simulink model "P6s"  (R2015b)
settings: Solver=VariableStepAuto  StartTime=0.0  StopTime=10.0  RelTol=1e-3
libraries: fl_lib x26, nesl_utility x9
settings Model: Creator=xmax1946  LastModifiedBy=xmax1946

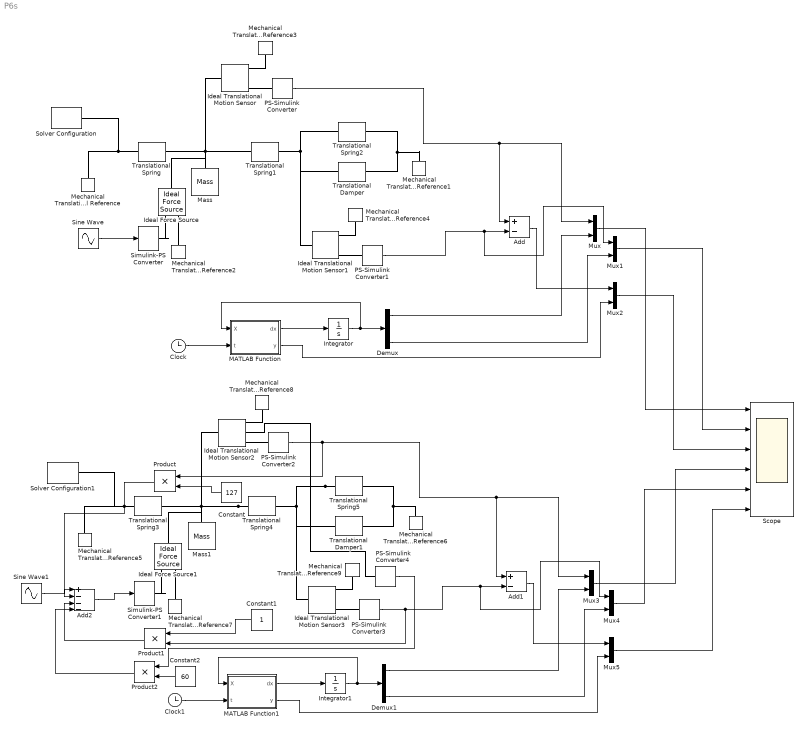
== system P6s ==
  Add : Sum  Inputs=+-
  Add1 : Sum  Inputs=+-
  Add2 : Sum  Inputs=+---
  Clock : Clock
  Clock1 : Clock
  Constant : Constant  Value=127
  Constant1 : Constant
  Constant2 : Constant  Value=60
  Demux : Demux  Outputs=3
  Demux1 : Demux  Outputs=3
  Ideal Force Source : fl_lib/Mechanical/Mechanical Sources/Ideal Force Source
  Ideal Force Source1 : fl_lib/Mechanical/Mechanical Sources/Ideal Force Source
  Ideal Translational Motion Sensor{,1..3} (4 alike) : fl_lib/Mechanical/Mechanical Sensors/Ideal Translational Motion Sensor  offset=0 m
  Integrator : Integrator  InitialCondition=[0;0;0]
  Integrator1 : Integrator  InitialCondition=[0;0;0]
  MATLAB Function : MATLAB Function  TreatAsAtomicUnit=on
  MATLAB Function1 : MATLAB Function  TreatAsAtomicUnit=on
  Mass : fl_lib/Mechanical/Translational Elements/Mass  mass=10 kg  v_specify=off  v_priority=None  v=0 m/s  f_specify=off  f_priority=None  f=0 N
  Mass1 : fl_lib/Mechanical/Translational Elements/Mass  mass=10 kg  v_specify=off  v_priority=None  v=0 m/s  f_specify=off  f_priority=None  f=0 N
  Mechanical Translational Reference{,1..9} (10 alike) : fl_lib/Mechanical/Translational Elements/Mechanical Translational Reference
  Mux{,1..5} (6 alike) : Mux  Inputs=2
  PS-Simulink Converter{,1..4} (5 alike) : nesl_utility/PS-Simulink Converter  PhysicalDomain=network_engine_domain  SubClassName=ps_output  LeftPortType=input  RightPortType=output  PseudoPeriodic=off  Frequencies=[]  Unit=1  AffineConversion=off
  Product : Product
  Product1 : Product
  Product2 : Product
  Scope : Scope  NumInputPorts=6
  Simulink-PS Converter : nesl_utility/Simulink-PS Converter  PhysicalDomain=network_engine_domain  SubClassName=ps_input  LeftPortType=input  RightPortType=output  PseudoPeriodic=off  Frequencies=[]  NoiseDistribution=none  NoiseParameters=[]  Unit=1  AffineConversion=off  InputFiltering=off  SimscapeFilterOrder=1  InputFilterTimeConstant=0.001  UdotUserProvided=1
  Simulink-PS Converter1 : nesl_utility/Simulink-PS Converter  PhysicalDomain=network_engine_domain  SubClassName=ps_input  LeftPortType=input  RightPortType=output  PseudoPeriodic=off  Frequencies=[]  NoiseDistribution=none  NoiseParameters=[]  Unit=1  AffineConversion=off  InputFiltering=off  SimscapeFilterOrder=1  InputFilterTimeConstant=0.001  UdotUserProvided=1
  Sine Wave : Sin  SampleTime=0
  Sine Wave1 : Sin  SampleTime=0
  Solver Configuration : nesl_utility/Solver Configuration  PhysicalDomain=network_engine_domain  SubClassName=solver  LeftPortType=input  RightPortType=generic  Accelerate=off  Tones=[]  Harmonics=[]  SimulateNoise=off  Profile=off  UseLocalSampling=off  EnableSwitchedLinearOptims=on  FrequencyDomain=off  UseCCode=off  RelTol=0.001  AbsTol=1e-06  MinStep=1e-09  ToWorkspace=off  RevertToSquareIcSolve=off  NumHomotopyIterations=100  PhasorMode=off  PhasorModeNumHarmonics=1  DoDC=off  ResidualTolerance=1e-09  UseLocalSolver=off  LocalSolverChoice=NE_BACKWARD_EULER_ADVANCER  LocalSolverSampleTime=0.001  DoFixedCost=off  MaxNonlinIter=3  MaxModeIter=2  LinearAlgebra=Sparse  DelaysMemoryBudget=1024  AutomaticFiltering=on  FilteringTimeConstant=0.001
  Solver Configuration1 : nesl_utility/Solver Configuration  PhysicalDomain=network_engine_domain  SubClassName=solver  LeftPortType=input  RightPortType=generic  Accelerate=off  Tones=[]  Harmonics=[]  SimulateNoise=off  Profile=off  UseLocalSampling=off  EnableSwitchedLinearOptims=on  FrequencyDomain=off  UseCCode=off  RelTol=0.001  AbsTol=1e-06  MinStep=1e-09  ToWorkspace=off  RevertToSquareIcSolve=off  NumHomotopyIterations=100  PhasorMode=off  PhasorModeNumHarmonics=1  DoDC=off  ResidualTolerance=1e-09  UseLocalSolver=off  LocalSolverChoice=NE_BACKWARD_EULER_ADVANCER  LocalSolverSampleTime=0.001  DoFixedCost=off  MaxNonlinIter=3  MaxModeIter=2  LinearAlgebra=Sparse  DelaysMemoryBudget=1024  AutomaticFiltering=on  FilteringTimeConstant=0.001
  Translational Damper : fl_lib/Mechanical/Translational Elements/Translational Damper  D=.5 N/(m/s)  v_specify=off  v_priority=None  v=0 m/s  f_specify=off  f_priority=None  f=0 N
  Translational Damper1 : fl_lib/Mechanical/Translational Elements/Translational Damper  D=.5 N/(m/s)  v_specify=off  v_priority=None  v=0 m/s  f_specify=off  f_priority=None  f=0 N
  Translational Spring : fl_lib/Mechanical/Translational Elements/Translational Spring  spr_rate=2 N/m  v_specify=off  v_priority=None  v=0 m/s  f_specify=off  f_priority=None  f=0 N  x_specify=off  x_priority=None  x=0 m
  Translational Spring1 : fl_lib/Mechanical/Translational Elements/Translational Spring  spr_rate=1 N/m  v_specify=off  v_priority=None  v=0 m/s  f_specify=off  f_priority=None  f=0 N  x_specify=off  x_priority=None  x=0 m
  Translational Spring2 : fl_lib/Mechanical/Translational Elements/Translational Spring  spr_rate=.5 N/m  v_specify=off  v_priority=None  v=0 m/s  f_specify=off  f_priority=None  f=0 N  x_specify=off  x_priority=None  x=0 m
  Translational Spring3 : fl_lib/Mechanical/Translational Elements/Translational Spring  spr_rate=2 N/m  v_specify=off  v_priority=None  v=0 m/s  f_specify=off  f_priority=None  f=0 N  x_specify=off  x_priority=None  x=0 m
  Translational Spring4 : fl_lib/Mechanical/Translational Elements/Translational Spring  spr_rate=1 N/m  v_specify=off  v_priority=None  v=0 m/s  f_specify=off  f_priority=None  f=0 N  x_specify=off  x_priority=None  x=0 m
  Translational Spring5 : fl_lib/Mechanical/Translational Elements/Translational Spring  spr_rate=.5 N/m  v_specify=off  v_priority=None  v=0 m/s  f_specify=off  f_priority=None  f=0 N  x_specify=off  x_priority=None  x=0 m
  wires:
  Sine Wave/1 -> Simulink-PS Converter/1
  PS-Simulink Converter/1 -> Mux/1, Add/1
  PS-Simulink Converter1/1 -> Mux1/1, Add/2
  MATLAB Function/1(dx) -> Integrator/1
  Integrator/1 -> MATLAB Function/1(X), Demux/1
  Clock/1 -> MATLAB Function/2(t)
  Mux/1 -> Scope/1
  Demux/1 -> Mux/2
  Mux1/1 -> Scope/2
  Demux/3 -> Mux1/2
  Mux2/1 -> Scope/3
  Add/1 -> Mux2/1
  MATLAB Function/2(y) -> Mux2/2
  PS-Simulink Converter3/1 -> Product1/2, Mux4/1, Add1/2
  MATLAB Function1/1(dx) -> Integrator1/1
  Integrator1/1 -> MATLAB Function1/1(X), Demux1/1
  Clock1/1 -> MATLAB Function1/2(t)
  Mux3/1 -> Scope/4
  Demux1/1 -> Mux3/2
  Mux4/1 -> Scope/5
  Demux1/3 -> Mux4/2
  Mux5/1 -> Scope/6
  Add1/1 -> Mux5/1
  MATLAB Function1/2(y) -> Mux5/2
  PS-Simulink Converter2/1 -> Product/1, Mux3/1, Add1/1
  Constant/1 -> Product/2
  Constant1/1 -> Product1/1
  Sine Wave1/1 -> Add2/1
  Product/1 -> Add2/2
  Product1/1 -> Add2/3
  Add2/1 -> Simulink-PS Converter1/1
  Constant2/1 -> Product2/2
  PS-Simulink Converter4/1 -> Product2/1
  Product2/1 -> Add2/4
  connections:
  Translational Spring/RConn1 -- Ideal Translational Motion Sensor/LConn1 -- Ideal Force Source/LConn1 -- Mass/LConn1 -- Translational Spring1/LConn1
  Translational Spring1/RConn1 -- Ideal Translational Motion Sensor1/LConn1 -- Translational Damper/LConn1 -- Translational Spring2/LConn1
  Mechanical Translational Reference/LConn1 -- Solver Configuration/RConn1 -- Translational Spring/LConn1
  Mechanical Translational Reference1/LConn1 -- Translational Spring2/RConn1 -- Translational Damper/RConn1
  Simulink-PS Converter/RConn1 -- Ideal Force Source/RConn1
  Mechanical Translational Reference2/LConn1 -- Ideal Force Source/RConn2
  Mechanical Translational Reference3/LConn1 -- Ideal Translational Motion Sensor/RConn1
  PS-Simulink Converter/LConn1 -- Ideal Translational Motion Sensor/RConn3
  PS-Simulink Converter1/LConn1 -- Ideal Translational Motion Sensor1/RConn3
  Mechanical Translational Reference4/LConn1 -- Ideal Translational Motion Sensor1/RConn1
  Translational Spring4/LConn1 -- Translational Spring3/RConn1 -- Ideal Translational Motion Sensor2/LConn1 -- Ideal Force Source1/LConn1 -- Mass1/LConn1
  Translational Spring5/LConn1 -- Translational Spring4/RConn1 -- Ideal Translational Motion Sensor3/LConn1 -- Translational Damper1/LConn1
  Translational Spring3/LConn1 -- Mechanical Translational Reference5/LConn1 -- Solver Configuration1/RConn1
  Translational Damper1/RConn1 -- Mechanical Translational Reference6/LConn1 -- Translational Spring5/RConn1
  Simulink-PS Converter1/RConn1 -- Ideal Force Source1/RConn1
  Mechanical Translational Reference7/LConn1 -- Ideal Force Source1/RConn2
  Mechanical Translational Reference8/LConn1 -- Ideal Translational Motion Sensor2/RConn1
  PS-Simulink Converter2/LConn1 -- Ideal Translational Motion Sensor2/RConn3
  PS-Simulink Converter3/LConn1 -- Ideal Translational Motion Sensor3/RConn3
  Mechanical Translational Reference9/LConn1 -- Ideal Translational Motion Sensor3/RConn1
  PS-Simulink Converter4/LConn1 -- Ideal Translational Motion Sensor2/RConn2

== matlab function P6s/MATLAB Function1 ==
  data: dx output; X input; y output; t input
function [dx,y] = fcn(X,t)

m1=10;
k1=2;
k2=1;
k3=.5;
b1=.5;
K=[127,60,1];
A=[0,1,0;-(k1+k2)/(m1),0,(k2)/(m1);(k2)/(b1),0,-(k2+k3)/(b1)];
B=[0;1/m1;0];
C=[1,0,-1];

u=sin(t)-K*X;

dx=A*X+B*u;
y=C*X;

== matlab function P6s/MATLAB Function ==
  data: dx output; X input; y output; t input
function [dx,y] = fcn(X,t)

m1=10;
k1=2;
k2=1;
k3=.5;
b1=.5;

A=[0,1,0;-(k1+k2)/(m1),0,(k2)/(m1);(k2)/(b1),0,-(k2+k3)/(b1)];
B=[0;1/m1;0];
C=[1,0,-1];
u=sin(t);
dx=A*X+B*u;
y=C*X;
